simulink model "LeftTrajectoryAgent"  (Simulink 6.5)
settings: Solver=ode45  SolverMode=SingleTasking  StartTime=0.0  StopTime=10.0  RelTol=1e-3  AbsTol=1e-6
settings Model: Creator=The MathWorks Inc.  LastModifiedBy=suarezjl  ExtModeTrigMode=oneshot  ExtModeArmWhenConnect=off  ExtModeAutoUpdateStatusClock=off
settings DataIOCC: LimitDataPoints=off  SignalLoggingName=logsOut
settings OptimizationCC: BooleanDataType=off  InlineInvariantSignals=on
settings DebuggingCC: CheckExecutionContextPreStartOutputMsg=on  CheckExecutionContextRuntimeOutputMsg=on  SolverPrmCheckMsg=none  MultiTaskDSMMsg=warning  MultiTaskCondExecSysMsg=none  IntegerOverflowMsg=none  StrictBusMsg=None
settings HardwareCC: TargetUnknown=on
settings ModelReferenceCC: UpdateModelReferenceTargets=IfOutOfDate
settings RTWCC: IncludeERTFirstTime=on

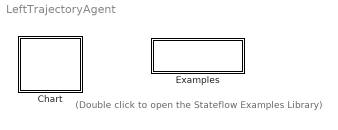
== system LeftTrajectoryAgent ==
  note: (Double click to open the
      | Stateflow Examples Library)
  Chart : Stateflow chart
  Examples : Subsystem
      settings: OpenFcn=sf('Private','sf_examples')
      mask Display: disp('Examples')

== system LeftTrajectoryAgent/Examples ==

== stateflow chart Chart ==
  state InitializeFunctions
    HungerForce\LeftReachDemo\LeftTrajectoryAgent\LoadHomePosition.Initialize()
    HungerForce\LeftReachDemo\LeftTrajectoryAgent\PlayCurrentTraj.Initialize()
    HungerForce\LeftReachDemo\LeftTrajectoryAgent\LoadHomePosition.Write2VS()
  state CopyCurrentLocation
    HungerForce\LeftReachDemo\LeftTrajectoryAgent\CopyGoalPosition.CopyRowVector()
    HungerForce\LeftReachDemo\LeftTrajectoryAgent\CopyCurrentPosition.CopyCurrentVector()
  state GenerateCurrentTrajectory
    HungerForce\LeftReachDemo\LeftTrajectoryAgent\GenerateCurrentTraj.GenerateTrajectory()
  state PlayCurrentTrajectory
    HungerForce\LeftReachDemo\LeftTrajectoryAgent\PlayCurrentTraj.OutputTrajectory()
    HungerForce\LeftReachDemo\LeftTrajectoryAgent\StateMachine.Wait(10000)
  state CopyHomeLocation
    HungerForce\LeftReachDemo\LeftTrajectoryAgent\CopyHomePosition.CopyRowVector()
    HungerForce\LeftReachDemo\LeftTrajectoryAgent\CopyCurrentPosition.CopyCurrentVector()
  state PlayHomeTrajectory
    HungerForce\LeftReachDemo\LeftTrajectoryAgent\PlayCurrentTraj.OutputTrajectory()
  state GenerateHomeTrajectory
    HungerForce\LeftReachDemo\LeftTrajectoryAgent\GenerateCurrentTraj.GenerateTrajectory()
  state Check that object is seen
    HungerForce\LeftReachDemo\LeftTrajectoryAgent\GenerateCurrentTraj.CheckForObject()
  (default) -> InitializeFunctions : Start
  InitializeFunctions -> Check that object is seen : Always
  CopyCurrentLocation -> GenerateCurrentTrajectory : Always
  GenerateCurrentTrajectory -> PlayCurrentTrajectory : Always
  PlayHomeTrajectory -> CopyCurrentLocation : Signal="Next"
  PlayCurrentTrajectory -> CopyHomeLocation : Always
  GenerateHomeTrajectory -> PlayHomeTrajectory : Signal="Next"
  CopyHomeLocation -> GenerateHomeTrajectory : Always
  Check that object is seen -> CopyCurrentLocation : Signal ="Next"
